simulink model "chase_high"  (R2016b)
settings: Solver=VariableStepAuto  StartTime=0.0  StopTime=10  FixedStep=0.01  MaxStep=1.0  RelTol=1e-3
settings Model: Creator=10448  LastModifiedBy=10448
settings ModelReferenceCC: ModelReferenceMinAlgLoopOccurrences=on

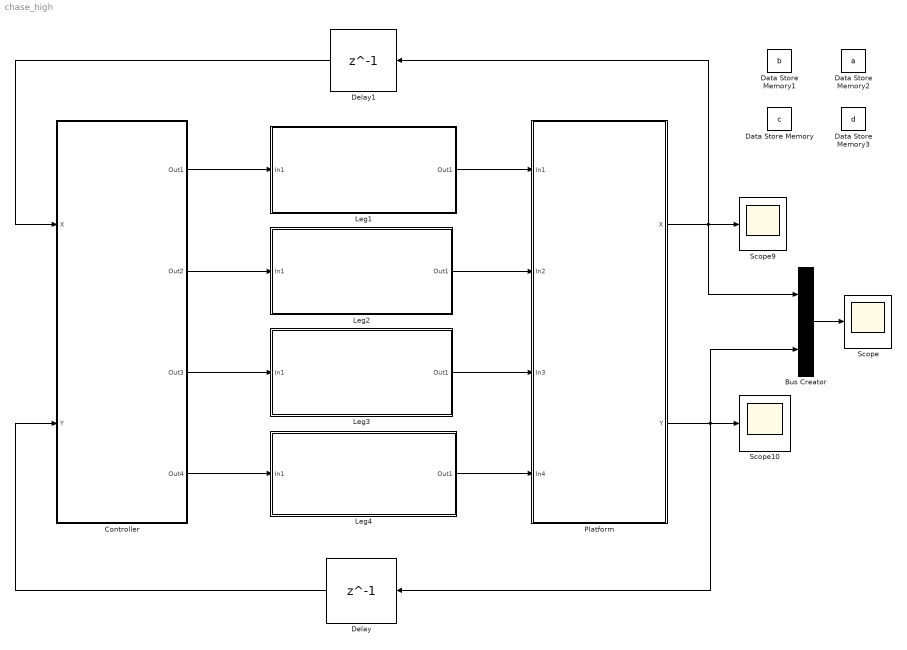
== system chase_high ==
  Bus Creator : BusCreator  Inputs=2
  Controller : Subsystem  TreatAsAtomicUnit=on
  Data Store Memory : DataStoreMemory  DataStoreName=c  ReadBeforeWriteMsg=warning  WriteAfterWriteMsg=warning  WriteAfterReadMsg=warning  InitialValue=245  ShowAdditionalParam=off  OutDataTypeStr=double
  Data Store Memory1 : DataStoreMemory  DataStoreName=b  ReadBeforeWriteMsg=warning  WriteAfterWriteMsg=warning  WriteAfterReadMsg=warning  InitialValue=230  ShowAdditionalParam=off  OutDataTypeStr=double
  Data Store Memory2 : DataStoreMemory  DataStoreName=a  ReadBeforeWriteMsg=warning  WriteAfterWriteMsg=warning  WriteAfterReadMsg=warning  InitialValue=240  ShowAdditionalParam=off  OutDataTypeStr=double
  Data Store Memory3 : DataStoreMemory  DataStoreName=d  ReadBeforeWriteMsg=warning  WriteAfterWriteMsg=warning  WriteAfterReadMsg=warning  InitialValue=250  ShowAdditionalParam=off  OutDataTypeStr=double
  Delay : Delay  DelayLength=1  SampleTime=3/700
  Delay1 : Delay  DelayLength=1  SampleTime=3/700
  Leg1 : Subsystem  TreatAsAtomicUnit=on
  Leg2 : Subsystem  TreatAsAtomicUnit=on
  Leg3 : Subsystem  TreatAsAtomicUnit=on
  Leg4 : Subsystem  TreatAsAtomicUnit=on
  Platform : Subsystem  TreatAsAtomicUnit=on
  Scope : Scope
  Scope10 : Scope
  Scope9 : Scope
  wires:
  Leg1/1(Out1) -> Platform/1(In1)
  Leg2/1(Out1) -> Platform/2(In2)
  Leg3/1(Out1) -> Platform/3(In3)
  Leg4/1(Out1) -> Platform/4(In4)
  Platform/1(X) -> Bus Creator/1, Scope9/1, Delay1/1
  Platform/2(Y) -> Delay/1, Scope10/1, Bus Creator/2
  Bus Creator/1 -> Scope/1
  Delay1/1 -> Controller/1(X)
  Delay/1 -> Controller/2(Y)
  Controller/1(Out1) -> Leg1/1(In1)
  Controller/2(Out2) -> Leg2/1(In1)
  Controller/3(Out3) -> Leg3/1(In1)
  Controller/4(Out4) -> Leg4/1(In1)

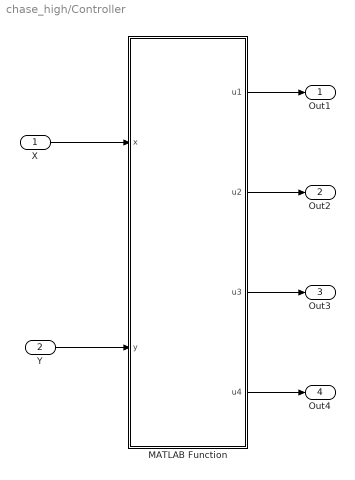
== system chase_high/Controller ==
  X : Inport
  Y : Inport  Port=2
  MATLAB Function : MATLAB Function  TreatAsAtomicUnit=on
  Out1 : Outport
  Out2 : Outport  Port=2
  Out3 : Outport  Port=3
  Out4 : Outport  Port=4
  wires:
  X/1 -> MATLAB Function/1(x)
  Y/1 -> MATLAB Function/2(y)
  MATLAB Function/1(u1) -> Out1/1
  MATLAB Function/2(u2) -> Out2/1
  MATLAB Function/3(u3) -> Out3/1
  MATLAB Function/4(u4) -> Out4/1

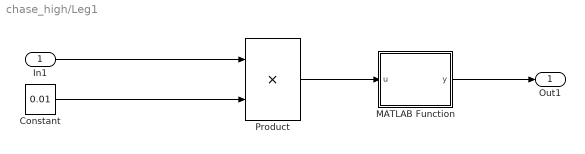
== system chase_high/Leg1 ==
  In1 : Inport
  Constant : Constant  Value=0.01
  MATLAB Function : MATLAB Function  TreatAsAtomicUnit=on
  Product : Product
  Out1 : Outport
  wires:
  MATLAB Function/1(y) -> Out1/1
  Constant/1 -> Product/2
  Product/1 -> MATLAB Function/1(u)
  In1/1 -> Product/1

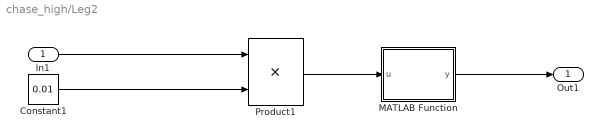
== system chase_high/Leg2 ==
  In1 : Inport
  Constant1 : Constant  Value=0.01
  MATLAB Function : MATLAB Function  TreatAsAtomicUnit=on
  Product1 : Product
  Out1 : Outport
  wires:
  MATLAB Function/1(y) -> Out1/1
  Constant1/1 -> Product1/2
  Product1/1 -> MATLAB Function/1(u)
  In1/1 -> Product1/1

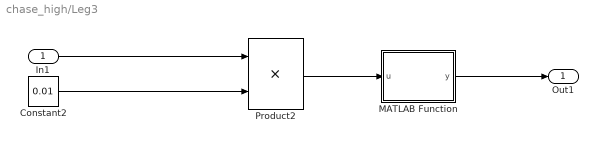
== system chase_high/Leg3 ==
  In1 : Inport
  Constant2 : Constant  Value=0.01
  MATLAB Function : MATLAB Function  TreatAsAtomicUnit=on
  Product2 : Product
  Out1 : Outport
  wires:
  MATLAB Function/1(y) -> Out1/1
  Constant2/1 -> Product2/2
  Product2/1 -> MATLAB Function/1(u)
  In1/1 -> Product2/1

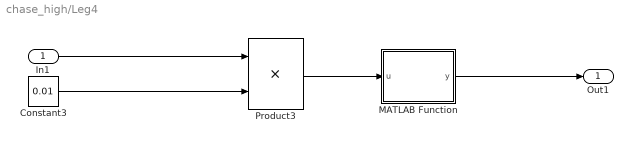
== system chase_high/Leg4 ==
  In1 : Inport
  Constant3 : Constant  Value=0.01
  MATLAB Function : MATLAB Function  TreatAsAtomicUnit=on
  Product3 : Product
  Out1 : Outport
  wires:
  MATLAB Function/1(y) -> Out1/1
  Product3/1 -> MATLAB Function/1(u)
  Constant3/1 -> Product3/2
  In1/1 -> Product3/1

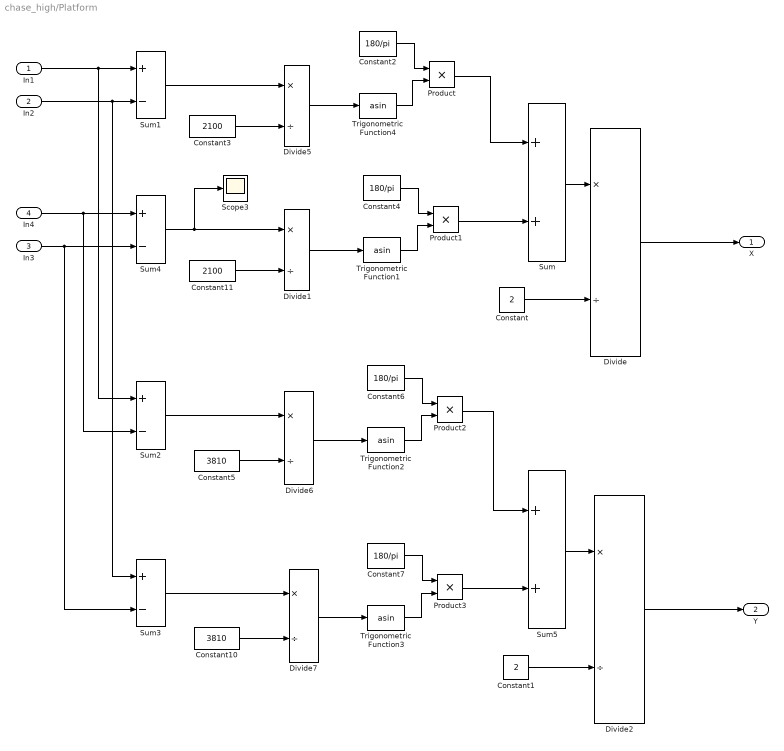
== system chase_high/Platform ==
  In1 : Inport
  In2 : Inport  Port=2
  In3 : Inport  Port=3
  In4 : Inport  Port=4
  Constant : Constant  Value=2
  Constant1 : Constant  Value=2
  Constant10 : Constant  Value=3810
  Constant11 : Constant  Value=2100
  Constant{2,4,6..7} (4 alike) : Constant  Value=180/pi
  Constant3 : Constant  Value=2100
  Constant5 : Constant  Value=3810
  Divide{,1..2,5..7} (6 alike) : Product  Inputs=*/
  Product{,1..3} (4 alike) : Product
  Scope3 : Scope
  Sum : Sum
  Sum{1..4} (4 alike) : Sum  Inputs=+-
  Sum5 : Sum
  Trigonometric Function{1..4} (4 alike) : Trigonometry  Operator=asin
  X : Outport
  Y : Outport  Port=2
  wires:
  Constant11/1 -> Divide1/2
  Sum4/1 -> Scope3/1, Divide1/1
  Constant3/1 -> Divide5/2
  Sum1/1 -> Divide5/1
  Constant5/1 -> Divide6/2
  Sum2/1 -> Divide6/1
  Constant10/1 -> Divide7/2
  Sum3/1 -> Divide7/1
  In1/1 -> Sum2/1, Sum1/1
  In2/1 -> Sum3/1, Sum1/2
  In4/1 -> Sum2/2, Sum4/1
  In3/1 -> Sum3/2, Sum4/2
  Sum/1 -> Divide/1
  Constant/1 -> Divide/2
  Sum5/1 -> Divide2/1
  Constant1/1 -> Divide2/2
  Divide/1 -> X/1
  Divide2/1 -> Y/1
  Divide5/1 -> Trigonometric Function4/1
  Constant2/1 -> Product/1
  Trigonometric Function4/1 -> Product/2
  Product/1 -> Sum/1
  Divide1/1 -> Trigonometric Function1/1
  Constant4/1 -> Product1/1
  Trigonometric Function1/1 -> Product1/2
  Product1/1 -> Sum/2
  Divide6/1 -> Trigonometric Function2/1
  Constant6/1 -> Product2/1
  Trigonometric Function2/1 -> Product2/2
  Product2/1 -> Sum5/1
  Divide7/1 -> Trigonometric Function3/1
  Constant7/1 -> Product3/1
  Trigonometric Function3/1 -> Product3/2
  Product3/1 -> Sum5/2

== matlab function chase_high/Leg3/MATLAB Function ==
  data: u input; y output; c data_store_memory
function y = fcn(u)
global c;
c= u+c;
y=c;

== matlab function chase_high/Controller/MATLAB Function ==
  data: x input; u1 output; y input; u2 output; u3 output; u4 output
function [u1,u2,u3,u4]= fcn(x,y)
if x>0.02&&y>0.02
    u3=1;u1=0;u2=0;u4=0;
else
    if x<-0.02&&y>0.02
        u4=1;u3=0;u1=0;u2=0;
    else
        if x<-0.02&&y<-0.02
            u1=1;u3=0;u2=0;u4=0;
        else
            if x>0.02&&y<-0.02
                u2=1;u3=0;u1=0;u4=0;
            else
                u1=0;u2=0;u3=0;u4=0;
            end
        end
    end
end
if (x>-0.02&&x<0.02)&&y>0.02
    u3=1;u4=1;u1=0;u2=0;
else
    if (x>-0.02&&x<0.02)&&y<-0.02
        u1=1;u2=1;u3=0;u4=0;
    else
        if x>0.02&&(y>-0.02&&y<0.02)
            u2=1;u3=1;u1=0;u4=0;
        else
            if x<-0.02&&(y>-0.02&&y<0.02)
                u1=1;u4=1;u3=0;u2=0;
            end
        end
    end
end

== matlab function chase_high/Leg2/MATLAB Function ==
  data: u input; y output; c data_store_memory; b data_store_memory
function y = fcn(u)
global b;
b= u+b;
y=b;

== matlab function chase_high/Leg1/MATLAB Function ==
  data: u input; y output; c data_store_memory; b data_store_memory; a data_store_memory
function y = fcn(u)
global a;
a= u+a;
y=a;

== matlab function chase_high/Leg4/MATLAB Function ==
  data: u input; y output; c data_store_memory; d data_store_memory
function y = fcn(u)
global d;
d= u+d;
y=d;
